simulink model "DFADAS2_SenFus_v1_201204RC_training_210115"  (R2018b)
settings: Solver=FixedStepDiscrete  StartTime=0.0  StopTime=inf  FixedStep=0.002  RelTol=1e-3  EnableMultiTasking=on
PreLoadFcn:
  | RTWConfigurationCB('preloadfcn', bdroot);
libraries: canmsglib x108, simulink x48, canfdmsglib x12
(part 5 of 28)

== system DFADAS2_SenFus_v1_201204RC_training_210115/Measure Calibration Debug/CAN Monitor (CANMon)/Subsystem1 ==
  <RLObj2> : Inport
  Bus Selector2 : BusSelector  OutputSignals=ID,Xpos,Ypos
  CAN Pack7 : canmsglib/CAN Pack  MsgList=(none)  MsgName=CAN Msg  MsgIDType=Standard (11-bit identifier)  MsgIdentifier=2033  MsgLength=8  SignalInfo=ID$0$16$1$2$1$0$1$0$-Inf$Inf$#Xpos$16$16$1$2$1$0$0.05$-400$-Inf$Inf$#Ypos$32$16$1$2$1$0$0.01$-80$-Inf$Inf$#  NSignals=3  StartBits=str2num('[int32(0);int32(16);int32(32)]')  SignalSizes=str2num('[int32(16);int32(16);int32(16)]')  ByteOrders=str2num('[int32(1);int32(1);int32(1)]')  DataTypes=str2num('[int32(2);int32(2);int32(2)]')  MultiplexTypes=str2num('[int32(1);int32(1);int32(1)]')  MultiplexValues=str2num('[double(0);double(0);double(0)]')  Factors=str2num('[double(1);double(0.05);double(0.01)]')  Offsets=str2num('[double(0);double(-400);double(-80)]')  Minimums=str2num('[double(-Inf);double(-Inf);double(-Inf)]')  Maximums=str2num('[double(Inf);double(Inf);double(Inf)]')  Remote=off  ApplyMinMax=off  BusOutput=on
      settings: SourceProductName=Simulink Real-Time  SourceProductBaseCode=XP  DataFormat=manually specified signals
  S-Function6 : S-Function  FunctionName=NSTC297CANTransmitBlkLib  Parameters=|  SFunctionDeploymentMode=off  EnableBusSupport=off  mask(NSTC297 CAN Transmit){Ns_DeviceID=General Control Unit Gen2, Ns_ChannelNum=0, Ns_FrameType=CAN, Ns_FrameBufferSize=0, Ns_OverflowCntOutFlg=off, Ns_SampleTime=-1}
      | uint16(Ns_DeviceID),
      | uint16(Ns_ChannelNum),
      | uint16(Ns_FrameType),
      | uint16(Ns_FrameBufferSize),
      | uint8(Ns_OverflowCntOutFlg),
      | double(Ns_SampleTime)
      mask prompts: Ns_DeviceID "Device:"; Ns_ChannelNum "Channel number:"; Ns_FrameType "Frame type:"; Ns_FrameBufferSize "Frame buffer size:"; Ns_OverflowCntOutFlg "Overflow count output"; Ns_SampleTime "Sample time:"
      mask init:
      | NSTC297CANTransmit_callback('portlabels');
      mask TypeOptions Ns_DeviceID: General Control Unit Gen2 | ADAS Control Unit Gen2
      mask TypeOptions Ns_ChannelNum: 0 | 1 | 2 | 3 | 4 | 5
      mask TypeOptions Ns_FrameType: CAN | CANFD
      mask Display: color('blue');text(0.98,0.9,'NovSteeds TC297','horizontalAlignment','right');color('blue');text(0.5,0.65,'CAN Transmit','horizontalAlignment','center');color('black');text(0.5,0.35,'Type: CAN','horizontalAlignment','center');text(0.5,0.50,'Channel: 0','horizontalAlignment','center');port_label('input',1, 'Msg');
  wires:
  CAN Pack7/1 -> S-Function6/1
  <RLObj2>/1 -> Bus Selector2/1
  Bus Selector2/2 -> CAN Pack7/2  "<Xpos>"
  Bus Selector2/3 -> CAN Pack7/3  "<Ypos>"
  Bus Selector2/1 -> CAN Pack7/1  "<ID>"

== system DFADAS2_SenFus_v1_201204RC_training_210115/Measure Calibration Debug/CAN Monitor (CANMon)/Subsystem2 ==
  <RLObj3> : Inport
  Bus Selector2 : BusSelector  OutputSignals=ID,Xpos,Ypos
  CAN Pack7 : canmsglib/CAN Pack  MsgList=(none)  MsgName=CAN Msg  MsgIDType=Standard (11-bit identifier)  MsgIdentifier=2034  MsgLength=8  SignalInfo=ID$0$16$1$2$1$0$1$0$-Inf$Inf$#Xpos$16$16$1$2$1$0$0.05$-400$-Inf$Inf$#Ypos$32$16$1$2$1$0$0.01$-80$-Inf$Inf$#  NSignals=3  StartBits=str2num('[int32(0);int32(16);int32(32)]')  SignalSizes=str2num('[int32(16);int32(16);int32(16)]')  ByteOrders=str2num('[int32(1);int32(1);int32(1)]')  DataTypes=str2num('[int32(2);int32(2);int32(2)]')  MultiplexTypes=str2num('[int32(1);int32(1);int32(1)]')  MultiplexValues=str2num('[double(0);double(0);double(0)]')  Factors=str2num('[double(1);double(0.05);double(0.01)]')  Offsets=str2num('[double(0);double(-400);double(-80)]')  Minimums=str2num('[double(-Inf);double(-Inf);double(-Inf)]')  Maximums=str2num('[double(Inf);double(Inf);double(Inf)]')  Remote=off  ApplyMinMax=off  BusOutput=on
      settings: SourceProductName=Simulink Real-Time  SourceProductBaseCode=XP  DataFormat=manually specified signals
  S-Function6 : S-Function  FunctionName=NSTC297CANTransmitBlkLib  Parameters=|  SFunctionDeploymentMode=off  EnableBusSupport=off  mask(NSTC297 CAN Transmit){Ns_DeviceID=General Control Unit Gen2, Ns_ChannelNum=0, Ns_FrameType=CAN, Ns_FrameBufferSize=0, Ns_OverflowCntOutFlg=off, Ns_SampleTime=-1}
      | uint16(Ns_DeviceID),
      | uint16(Ns_ChannelNum),
      | uint16(Ns_FrameType),
      | uint16(Ns_FrameBufferSize),
      | uint8(Ns_OverflowCntOutFlg),
      | double(Ns_SampleTime)
      mask prompts: Ns_DeviceID "Device:"; Ns_ChannelNum "Channel number:"; Ns_FrameType "Frame type:"; Ns_FrameBufferSize "Frame buffer size:"; Ns_OverflowCntOutFlg "Overflow count output"; Ns_SampleTime "Sample time:"
      mask init:
      | NSTC297CANTransmit_callback('portlabels');
      mask TypeOptions Ns_DeviceID: General Control Unit Gen2 | ADAS Control Unit Gen2
      mask TypeOptions Ns_ChannelNum: 0 | 1 | 2 | 3 | 4 | 5
      mask TypeOptions Ns_FrameType: CAN | CANFD
      mask Display: color('blue');text(0.98,0.9,'NovSteeds TC297','horizontalAlignment','right');color('blue');text(0.5,0.65,'CAN Transmit','horizontalAlignment','center');color('black');text(0.5,0.35,'Type: CAN','horizontalAlignment','center');text(0.5,0.50,'Channel: 0','horizontalAlignment','center');port_label('input',1, 'Msg');
  wires:
  CAN Pack7/1 -> S-Function6/1
  <RLObj3>/1 -> Bus Selector2/1
  Bus Selector2/2 -> CAN Pack7/2  "<Xpos>"
  Bus Selector2/3 -> CAN Pack7/3  "<Ypos>"
  Bus Selector2/1 -> CAN Pack7/1  "<ID>"

== system DFADAS2_SenFus_v1_201204RC_training_210115/Measure Calibration Debug/CAN Monitor (CANMon)/Subsystem3 ==
  <RLObj4> : Inport
  Bus Selector2 : BusSelector  OutputSignals=ID,Xpos,Ypos
  CAN Pack7 : canmsglib/CAN Pack  MsgList=(none)  MsgName=CAN Msg  MsgIDType=Standard (11-bit identifier)  MsgIdentifier=2035  MsgLength=8  SignalInfo=ID$0$16$1$2$1$0$1$0$-Inf$Inf$#Xpos$16$16$1$2$1$0$0.05$-400$-Inf$Inf$#Ypos$32$16$1$2$1$0$0.01$-80$-Inf$Inf$#  NSignals=3  StartBits=str2num('[int32(0);int32(16);int32(32)]')  SignalSizes=str2num('[int32(16);int32(16);int32(16)]')  ByteOrders=str2num('[int32(1);int32(1);int32(1)]')  DataTypes=str2num('[int32(2);int32(2);int32(2)]')  MultiplexTypes=str2num('[int32(1);int32(1);int32(1)]')  MultiplexValues=str2num('[double(0);double(0);double(0)]')  Factors=str2num('[double(1);double(0.05);double(0.01)]')  Offsets=str2num('[double(0);double(-400);double(-80)]')  Minimums=str2num('[double(-Inf);double(-Inf);double(-Inf)]')  Maximums=str2num('[double(Inf);double(Inf);double(Inf)]')  Remote=off  ApplyMinMax=off  BusOutput=on
      settings: SourceProductName=Simulink Real-Time  SourceProductBaseCode=XP  DataFormat=manually specified signals
  S-Function6 : S-Function  FunctionName=NSTC297CANTransmitBlkLib  Parameters=|  SFunctionDeploymentMode=off  EnableBusSupport=off  mask(NSTC297 CAN Transmit){Ns_DeviceID=General Control Unit Gen2, Ns_ChannelNum=0, Ns_FrameType=CAN, Ns_FrameBufferSize=0, Ns_OverflowCntOutFlg=off, Ns_SampleTime=-1}
      | uint16(Ns_DeviceID),
      | uint16(Ns_ChannelNum),
      | uint16(Ns_FrameType),
      | uint16(Ns_FrameBufferSize),
      | uint8(Ns_OverflowCntOutFlg),
      | double(Ns_SampleTime)
      mask prompts: Ns_DeviceID "Device:"; Ns_ChannelNum "Channel number:"; Ns_FrameType "Frame type:"; Ns_FrameBufferSize "Frame buffer size:"; Ns_OverflowCntOutFlg "Overflow count output"; Ns_SampleTime "Sample time:"
      mask init:
      | NSTC297CANTransmit_callback('portlabels');
      mask TypeOptions Ns_DeviceID: General Control Unit Gen2 | ADAS Control Unit Gen2
      mask TypeOptions Ns_ChannelNum: 0 | 1 | 2 | 3 | 4 | 5
      mask TypeOptions Ns_FrameType: CAN | CANFD
      mask Display: color('blue');text(0.98,0.9,'NovSteeds TC297','horizontalAlignment','right');color('blue');text(0.5,0.65,'CAN Transmit','horizontalAlignment','center');color('black');text(0.5,0.35,'Type: CAN','horizontalAlignment','center');text(0.5,0.50,'Channel: 0','horizontalAlignment','center');port_label('input',1, 'Msg');
  wires:
  Bus Selector2/1 -> CAN Pack7/1  "<ID>"
  Bus Selector2/3 -> CAN Pack7/3  "<Ypos>"
  Bus Selector2/2 -> CAN Pack7/2  "<Xpos>"
  <RLObj4>/1 -> Bus Selector2/1
  CAN Pack7/1 -> S-Function6/1

== system DFADAS2_SenFus_v1_201204RC_training_210115/Measure Calibration Debug/CAN Monitor (CANMon)/Subsystem4 ==
  <RLObj5> : Inport
  Bus Selector2 : BusSelector  OutputSignals=ID,Xpos,Ypos
  CAN Pack7 : canmsglib/CAN Pack  MsgList=(none)  MsgName=CAN Msg  MsgIDType=Standard (11-bit identifier)  MsgIdentifier=2036  MsgLength=8  SignalInfo=ID$0$16$1$2$1$0$1$0$-Inf$Inf$#Xpos$16$16$1$2$1$0$0.05$-400$-Inf$Inf$#Ypos$32$16$1$2$1$0$0.01$-80$-Inf$Inf$#  NSignals=3  StartBits=str2num('[int32(0);int32(16);int32(32)]')  SignalSizes=str2num('[int32(16);int32(16);int32(16)]')  ByteOrders=str2num('[int32(1);int32(1);int32(1)]')  DataTypes=str2num('[int32(2);int32(2);int32(2)]')  MultiplexTypes=str2num('[int32(1);int32(1);int32(1)]')  MultiplexValues=str2num('[double(0);double(0);double(0)]')  Factors=str2num('[double(1);double(0.05);double(0.01)]')  Offsets=str2num('[double(0);double(-400);double(-80)]')  Minimums=str2num('[double(-Inf);double(-Inf);double(-Inf)]')  Maximums=str2num('[double(Inf);double(Inf);double(Inf)]')  Remote=off  ApplyMinMax=off  BusOutput=on
      settings: SourceProductName=Simulink Real-Time  SourceProductBaseCode=XP  DataFormat=manually specified signals
  S-Function6 : S-Function  FunctionName=NSTC297CANTransmitBlkLib  Parameters=|  SFunctionDeploymentMode=off  EnableBusSupport=off  mask(NSTC297 CAN Transmit){Ns_DeviceID=General Control Unit Gen2, Ns_ChannelNum=0, Ns_FrameType=CAN, Ns_FrameBufferSize=0, Ns_OverflowCntOutFlg=off, Ns_SampleTime=-1}
      | uint16(Ns_DeviceID),
      | uint16(Ns_ChannelNum),
      | uint16(Ns_FrameType),
      | uint16(Ns_FrameBufferSize),
      | uint8(Ns_OverflowCntOutFlg),
      | double(Ns_SampleTime)
      mask prompts: Ns_DeviceID "Device:"; Ns_ChannelNum "Channel number:"; Ns_FrameType "Frame type:"; Ns_FrameBufferSize "Frame buffer size:"; Ns_OverflowCntOutFlg "Overflow count output"; Ns_SampleTime "Sample time:"
      mask init:
      | NSTC297CANTransmit_callback('portlabels');
      mask TypeOptions Ns_DeviceID: General Control Unit Gen2 | ADAS Control Unit Gen2
      mask TypeOptions Ns_ChannelNum: 0 | 1 | 2 | 3 | 4 | 5
      mask TypeOptions Ns_FrameType: CAN | CANFD
      mask Display: color('blue');text(0.98,0.9,'NovSteeds TC297','horizontalAlignment','right');color('blue');text(0.5,0.65,'CAN Transmit','horizontalAlignment','center');color('black');text(0.5,0.35,'Type: CAN','horizontalAlignment','center');text(0.5,0.50,'Channel: 0','horizontalAlignment','center');port_label('input',1, 'Msg');
  wires:
  CAN Pack7/1 -> S-Function6/1
  <RLObj5>/1 -> Bus Selector2/1
  Bus Selector2/2 -> CAN Pack7/2  "<Xpos>"
  Bus Selector2/3 -> CAN Pack7/3  "<Ypos>"
  Bus Selector2/1 -> CAN Pack7/1  "<ID>"

== system DFADAS2_SenFus_v1_201204RC_training_210115/Measure Calibration Debug/CAN Monitor (CANMon)/Subsystem5 ==
  <RLObj6> : Inport
  Bus Selector2 : BusSelector  OutputSignals=ID,Xpos,Ypos
  CAN Pack7 : canmsglib/CAN Pack  MsgList=(none)  MsgName=CAN Msg  MsgIDType=Standard (11-bit identifier)  MsgIdentifier=2037  MsgLength=8  SignalInfo=ID$0$16$1$2$1$0$1$0$-Inf$Inf$#Xpos$16$16$1$2$1$0$0.05$-400$-Inf$Inf$#Ypos$32$16$1$2$1$0$0.01$-80$-Inf$Inf$#  NSignals=3  StartBits=str2num('[int32(0);int32(16);int32(32)]')  SignalSizes=str2num('[int32(16);int32(16);int32(16)]')  ByteOrders=str2num('[int32(1);int32(1);int32(1)]')  DataTypes=str2num('[int32(2);int32(2);int32(2)]')  MultiplexTypes=str2num('[int32(1);int32(1);int32(1)]')  MultiplexValues=str2num('[double(0);double(0);double(0)]')  Factors=str2num('[double(1);double(0.05);double(0.01)]')  Offsets=str2num('[double(0);double(-400);double(-80)]')  Minimums=str2num('[double(-Inf);double(-Inf);double(-Inf)]')  Maximums=str2num('[double(Inf);double(Inf);double(Inf)]')  Remote=off  ApplyMinMax=off  BusOutput=on
      settings: SourceProductName=Simulink Real-Time  SourceProductBaseCode=XP  DataFormat=manually specified signals
  S-Function6 : S-Function  FunctionName=NSTC297CANTransmitBlkLib  Parameters=|  SFunctionDeploymentMode=off  EnableBusSupport=off  mask(NSTC297 CAN Transmit){Ns_DeviceID=General Control Unit Gen2, Ns_ChannelNum=0, Ns_FrameType=CAN, Ns_FrameBufferSize=0, Ns_OverflowCntOutFlg=off, Ns_SampleTime=-1}
      | uint16(Ns_DeviceID),
      | uint16(Ns_ChannelNum),
      | uint16(Ns_FrameType),
      | uint16(Ns_FrameBufferSize),
      | uint8(Ns_OverflowCntOutFlg),
      | double(Ns_SampleTime)
      mask prompts: Ns_DeviceID "Device:"; Ns_ChannelNum "Channel number:"; Ns_FrameType "Frame type:"; Ns_FrameBufferSize "Frame buffer size:"; Ns_OverflowCntOutFlg "Overflow count output"; Ns_SampleTime "Sample time:"
      mask init:
      | NSTC297CANTransmit_callback('portlabels');
      mask TypeOptions Ns_DeviceID: General Control Unit Gen2 | ADAS Control Unit Gen2
      mask TypeOptions Ns_ChannelNum: 0 | 1 | 2 | 3 | 4 | 5
      mask TypeOptions Ns_FrameType: CAN | CANFD
      mask Display: color('blue');text(0.98,0.9,'NovSteeds TC297','horizontalAlignment','right');color('blue');text(0.5,0.65,'CAN Transmit','horizontalAlignment','center');color('black');text(0.5,0.35,'Type: CAN','horizontalAlignment','center');text(0.5,0.50,'Channel: 0','horizontalAlignment','center');port_label('input',1, 'Msg');
  wires:
  Bus Selector2/1 -> CAN Pack7/1  "<ID>"
  Bus Selector2/3 -> CAN Pack7/3  "<Ypos>"
  Bus Selector2/2 -> CAN Pack7/2  "<Xpos>"
  <RLObj6>/1 -> Bus Selector2/1
  CAN Pack7/1 -> S-Function6/1

== system DFADAS2_SenFus_v1_201204RC_training_210115/Measure Calibration Debug/CAN Monitor (CANMon)/Subsystem6 ==
  <RLObj7> : Inport
  Bus Selector2 : BusSelector  OutputSignals=ID,Xpos,Ypos
  CAN Pack7 : canmsglib/CAN Pack  MsgList=(none)  MsgName=CAN Msg  MsgIDType=Standard (11-bit identifier)  MsgIdentifier=2038  MsgLength=8  SignalInfo=ID$0$16$1$2$1$0$1$0$-Inf$Inf$#Xpos$16$16$1$2$1$0$0.05$-400$-Inf$Inf$#Ypos$32$16$1$2$1$0$0.01$-80$-Inf$Inf$#  NSignals=3  StartBits=str2num('[int32(0);int32(16);int32(32)]')  SignalSizes=str2num('[int32(16);int32(16);int32(16)]')  ByteOrders=str2num('[int32(1);int32(1);int32(1)]')  DataTypes=str2num('[int32(2);int32(2);int32(2)]')  MultiplexTypes=str2num('[int32(1);int32(1);int32(1)]')  MultiplexValues=str2num('[double(0);double(0);double(0)]')  Factors=str2num('[double(1);double(0.05);double(0.01)]')  Offsets=str2num('[double(0);double(-400);double(-80)]')  Minimums=str2num('[double(-Inf);double(-Inf);double(-Inf)]')  Maximums=str2num('[double(Inf);double(Inf);double(Inf)]')  Remote=off  ApplyMinMax=off  BusOutput=on
      settings: SourceProductName=Simulink Real-Time  SourceProductBaseCode=XP  DataFormat=manually specified signals
  S-Function6 : S-Function  FunctionName=NSTC297CANTransmitBlkLib  Parameters=|  SFunctionDeploymentMode=off  EnableBusSupport=off  mask(NSTC297 CAN Transmit){Ns_DeviceID=General Control Unit Gen2, Ns_ChannelNum=0, Ns_FrameType=CAN, Ns_FrameBufferSize=0, Ns_OverflowCntOutFlg=off, Ns_SampleTime=-1}
      | uint16(Ns_DeviceID),
      | uint16(Ns_ChannelNum),
      | uint16(Ns_FrameType),
      | uint16(Ns_FrameBufferSize),
      | uint8(Ns_OverflowCntOutFlg),
      | double(Ns_SampleTime)
      mask prompts: Ns_DeviceID "Device:"; Ns_ChannelNum "Channel number:"; Ns_FrameType "Frame type:"; Ns_FrameBufferSize "Frame buffer size:"; Ns_OverflowCntOutFlg "Overflow count output"; Ns_SampleTime "Sample time:"
      mask init:
      | NSTC297CANTransmit_callback('portlabels');
      mask TypeOptions Ns_DeviceID: General Control Unit Gen2 | ADAS Control Unit Gen2
      mask TypeOptions Ns_ChannelNum: 0 | 1 | 2 | 3 | 4 | 5
      mask TypeOptions Ns_FrameType: CAN | CANFD
      mask Display: color('blue');text(0.98,0.9,'NovSteeds TC297','horizontalAlignment','right');color('blue');text(0.5,0.65,'CAN Transmit','horizontalAlignment','center');color('black');text(0.5,0.35,'Type: CAN','horizontalAlignment','center');text(0.5,0.50,'Channel: 0','horizontalAlignment','center');port_label('input',1, 'Msg');
  wires:
  Bus Selector2/1 -> CAN Pack7/1  "<ID>"
  Bus Selector2/3 -> CAN Pack7/3  "<Ypos>"
  Bus Selector2/2 -> CAN Pack7/2  "<Xpos>"
  <RLObj7>/1 -> Bus Selector2/1
  CAN Pack7/1 -> S-Function6/1

== system DFADAS2_SenFus_v1_201204RC_training_210115/Measure Calibration Debug/CAN Monitor (CANMon)/Subsystem7 ==
  <RLObj8> : Inport
  Bus Selector2 : BusSelector  OutputSignals=ID,Xpos,Ypos
  CAN Pack7 : canmsglib/CAN Pack  MsgList=(none)  MsgName=CAN Msg  MsgIDType=Standard (11-bit identifier)  MsgIdentifier=2039  MsgLength=8  SignalInfo=ID$0$16$1$2$1$0$1$0$-Inf$Inf$#Xpos$16$16$1$2$1$0$0.05$-400$-Inf$Inf$#Ypos$32$16$1$2$1$0$0.01$-80$-Inf$Inf$#  NSignals=3  StartBits=str2num('[int32(0);int32(16);int32(32)]')  SignalSizes=str2num('[int32(16);int32(16);int32(16)]')  ByteOrders=str2num('[int32(1);int32(1);int32(1)]')  DataTypes=str2num('[int32(2);int32(2);int32(2)]')  MultiplexTypes=str2num('[int32(1);int32(1);int32(1)]')  MultiplexValues=str2num('[double(0);double(0);double(0)]')  Factors=str2num('[double(1);double(0.05);double(0.01)]')  Offsets=str2num('[double(0);double(-400);double(-80)]')  Minimums=str2num('[double(-Inf);double(-Inf);double(-Inf)]')  Maximums=str2num('[double(Inf);double(Inf);double(Inf)]')  Remote=off  ApplyMinMax=off  BusOutput=on
      settings: SourceProductName=Simulink Real-Time  SourceProductBaseCode=XP  DataFormat=manually specified signals
  S-Function6 : S-Function  FunctionName=NSTC297CANTransmitBlkLib  Parameters=|  SFunctionDeploymentMode=off  EnableBusSupport=off  mask(NSTC297 CAN Transmit){Ns_DeviceID=General Control Unit Gen2, Ns_ChannelNum=0, Ns_FrameType=CAN, Ns_FrameBufferSize=0, Ns_OverflowCntOutFlg=off, Ns_SampleTime=-1}
      | uint16(Ns_DeviceID),
      | uint16(Ns_ChannelNum),
      | uint16(Ns_FrameType),
      | uint16(Ns_FrameBufferSize),
      | uint8(Ns_OverflowCntOutFlg),
      | double(Ns_SampleTime)
      mask prompts: Ns_DeviceID "Device:"; Ns_ChannelNum "Channel number:"; Ns_FrameType "Frame type:"; Ns_FrameBufferSize "Frame buffer size:"; Ns_OverflowCntOutFlg "Overflow count output"; Ns_SampleTime "Sample time:"
      mask init:
      | NSTC297CANTransmit_callback('portlabels');
      mask TypeOptions Ns_DeviceID: General Control Unit Gen2 | ADAS Control Unit Gen2
      mask TypeOptions Ns_ChannelNum: 0 | 1 | 2 | 3 | 4 | 5
      mask TypeOptions Ns_FrameType: CAN | CANFD
      mask Display: color('blue');text(0.98,0.9,'NovSteeds TC297','horizontalAlignment','right');color('blue');text(0.5,0.65,'CAN Transmit','horizontalAlignment','center');color('black');text(0.5,0.35,'Type: CAN','horizontalAlignment','center');text(0.5,0.50,'Channel: 0','horizontalAlignment','center');port_label('input',1, 'Msg');
  wires:
  CAN Pack7/1 -> S-Function6/1
  <RLObj8>/1 -> Bus Selector2/1
  Bus Selector2/2 -> CAN Pack7/2  "<Xpos>"
  Bus Selector2/3 -> CAN Pack7/3  "<Ypos>"
  Bus Selector2/1 -> CAN Pack7/1  "<ID>"

== system DFADAS2_SenFus_v1_201204RC_training_210115/Signal Input (Input)/Signal Input (10ms) (Input10)/Others ==
  Bus Creator1 : BusCreator  Inputs=3
  Constant4 : Constant  Value=0.3
  Constant5 : Constant  Value=0.3
  Constant6 : Constant  Value=0.3
  Out1 : Outport
  wires:
  Bus Creator1/1 -> Out1/1  "VehInfo"
  Constant6/1 -> Bus Creator1/3
  Constant5/1 -> Bus Creator1/2
  Constant4/1 -> Bus Creator1/1

== system DFADAS2_SenFus_v1_201204RC_training_210115/Signal Input (Input)/Signal Input (10ms) (Input10)/VehInfo ==
  note: Level: 2
  ACC_AdditionalSignal_1 : Subsystem
  ACC_AdditionalSignal_20190523 : Subsystem
  Body Electric System State Receive and Processing (BESRx) : Subsystem
  Bus Creator2 : BusCreator  Inputs=10
  EPS Signal Receive and Processing (EPSRx) : Subsystem
  "ForwardVeh_sigback " : Subsystem
  From ACC (From ACC) : Subsystem
  Function Keys State Receive and Processing (FKeyStRx) : Subsystem
  MP5 Signal Receive (MP5Rx)1 : Subsystem
  Powertrain State Receive and Processing (PTRx) : Subsystem
  Steeing Wheel Angle Receive and Processing (SWARx) : Subsystem
  Vehicle Movement Signal Receive and Processing (VehMovRx) : Subsystem
  VehInfo : Outport
  tag scope: Acc_DisplaySig=global
  wires:
  Bus Creator2/1 -> VehInfo/1  "bsVehInfo"
  ACC_AdditionalSignal_1/1(Acc_DisplaySig) -> [Acc_DisplaySig]
  MP5 Signal Receive (MP5Rx)1/1(MP5Rx_bsMP5Info) -> Bus Creator2/1  "MP5Rx_bsMP5Info"
  EPS Signal Receive and Processing (EPSRx)/1(EPSRx_bsEPSInfo) -> Bus Creator2/2  "EPSRx_bsEPSInfo"
  Vehicle Movement Signal Receive and Processing (VehMovRx)/1(VehMovRx_bsVehMovInfo) -> Bus Creator2/3  "VehMovRx_bsVehMovInfo"
  Steeing Wheel Angle Receive and Processing (SWARx)/1(SWARx_bsSWAInfo) -> Bus Creator2/4  "SWARx_bsSWAInfo"
  Body Electric System State Receive and Processing (BESRx)/1(BESRx_bsBESState) -> Bus Creator2/5  "BESRx_bsBESState"
  Function Keys State Receive and Processing (FKeyStRx)/1(FKeyStRx_stFKeyState) -> Bus Creator2/6  "FKeyStRx_stFKeyState"
  Powertrain State Receive and Processing (PTRx)/1(PTRx_bsPTState) -> Bus Creator2/7  "PTRx_bsPTState"
  From ACC (From ACC)/1(From ACC_stACCState) -> Bus Creator2/8  "From ACC_stACCState"
  ACC_AdditionalSignal_20190523/1(DACIn_bsACCAdditionalSignal) -> Bus Creator2/9  "FMCRx_ACCAdditionalSignal"
  "ForwardVeh_sigback "/1(SpdReq_bsSpdDet1info) -> Bus Creator2/10  "SpdReq_bsSpdDet1info"

== system DFADAS2_SenFus_v1_201204RC_training_210115/Signal Input (Input)/Signal Input (50ms) (Input50)/Cmr ==
  note: Device Signal Level
  Camera Objects Information (CmrObjInfo) : Subsystem
  CmrInfo : Subsystem
  Cmr_bsComInfo : Outport
  Cmr_bsTrafSig : Outport  Port=2
  Cmr_bsObjInfo : Outport  Port=3
  wires:
  Camera Objects Information (CmrObjInfo)/1(CmrObjRx_bsObjInfo) -> Cmr_bsObjInfo/1  "CmrObjInfo"
  CmrInfo/1(LaneRx_bsLaneInfo) -> Cmr_bsComInfo/1  "LaneInfo"

== system DFADAS2_SenFus_v1_201204RC_training_210115/Signal Input (Input)/Signal Input (50ms) (Input50)/Front Left Radar(S2) Objects Information (FLRdr) ==
  Bus Creator : BusCreator  Inputs=2
  Bus Selector : BusSelector  OutputSignals=NumberOfObjects_S2
  Constant1 : Constant  SampleTime=0.05
  Constant2 : Constant  SampleTime=0.05
  Constant3 : Constant  SampleTime=0.05
  S0 Data Frame Read : Subsystem  TreatAsAtomicUnit=on
  S0 Header Frame Read : Subsystem  TreatAsAtomicUnit=on
  S0 Trailer Frame Read : Subsystem  TreatAsAtomicUnit=on
  Subsystem : Subsystem  Commented=on
  FLRdr_bsObjInfo : Outport
  wires:
  Bus Creator/1 -> FLRdr_bsObjInfo/1, Subsystem/1(In1)
  Bus Selector/1 -> S0 Data Frame Read/3(ObjectNum)  "<NumberOfObjects_S2>"
  S0 Header Frame Read/1(RLRdr_bsCmnInfo) -> Bus Selector/1, Bus Creator/1  "FLRdr_bsCmnInfo"
  S0 Data Frame Read/1(RLRdr_bsObjInfo) -> Bus Creator/2  "FLRdr_bsObjInfo"
  Constant2/1 -> S0 Data Frame Read/2(IC)
  Constant1/1 -> S0 Trailer Frame Read/2("IC ")
  Constant3/1 -> S0 Header Frame Read/1(IC)
  S0 Header Frame Read/2(HFVFCnt) -> S0 Data Frame Read/1(HFVFCnt), S0 Trailer Frame Read/1(HFVFCnt)

== system DFADAS2_SenFus_v1_201204RC_training_210115/Signal Input (Input)/Signal Input (50ms) (Input50)/Front Right Radar(S3) Objects Information (FRRdr) ==
  Bus Creator : BusCreator  Inputs=2
  Bus Selector : BusSelector  OutputSignals=NumberOfObjects_S3
  Constant1 : Constant  SampleTime=0.05
  Constant2 : Constant  SampleTime=0.05
  Constant3 : Constant  SampleTime=0.05
  S0 Data Frame Read : Subsystem  TreatAsAtomicUnit=on
  S0 Header Frame Read : Subsystem  TreatAsAtomicUnit=on
  S0 Trailer Frame Read : Subsystem  TreatAsAtomicUnit=on
  Subsystem : Subsystem  Commented=on
  FRRdr_bsObjInfo : Outport
  wires:
  Bus Creator/1 -> FRRdr_bsObjInfo/1, Subsystem/1(In1)
  S0 Data Frame Read/1(RLRdr_bsObjInfo) -> Bus Creator/2  "FRRdr_bsObjInfo"
  S0 Header Frame Read/2(HFVFCnt) -> S0 Trailer Frame Read/1(HFVFCnt), S0 Data Frame Read/1(HFVFCnt)
  Constant3/1 -> S0 Header Frame Read/1(IC)
  Constant1/1 -> S0 Trailer Frame Read/2("IC ")
  Constant2/1 -> S0 Data Frame Read/2(IC)
  S0 Header Frame Read/1(RLRdr_bsCmnInfo) -> Bus Selector/1, Bus Creator/1  "FRRdr_bsCmnInfo"
  Bus Selector/1 -> S0 Data Frame Read/3(ObjectNum)  "<NumberOfObjects_S3>"

== system DFADAS2_SenFus_v1_201204RC_training_210115/Signal Input (Input)/Signal Input (50ms) (Input50)/Others ==
  Bus Creator1 : BusCreator  Inputs=3
  Constant4 : Constant  Value=0.3
  Constant5 : Constant  Value=0.3
  Constant6 : Constant  Value=0.3
  Out1 : Outport
  wires:
  Bus Creator1/1 -> Out1/1  "VehInfo"
  Constant6/1 -> Bus Creator1/3
  Constant5/1 -> Bus Creator1/2
  Constant4/1 -> Bus Creator1/1

== system DFADAS2_SenFus_v1_201204RC_training_210115/Signal Input (Input)/Signal Input (50ms) (Input50)/RdrFrt ==
  note: ① 设备：完整性
      | ② 信号及状态
  note: 首先按设备分层；然后按功能对信号聚类与分层。
  Bus Creator1 : BusCreator  Inputs=2
  CmrInfo : Subsystem
  Rdr1 : Subsystem
  Out1 : Outport
  wires:
  Bus Creator1/1 -> Out1/1
  Rdr1/1(Out1) -> Bus Creator1/2
  CmrInfo/1(Out1) -> Bus Creator1/1

== system DFADAS2_SenFus_v1_201204RC_training_210115/Signal Input (Input)/Signal Input (50ms) (Input50)/Rear Left Radar(S0) Objects Information (RLRdr) ==
  Bus Creator : BusCreator  Inputs=2
  Bus Selector : BusSelector  OutputSignals=NumberOfObjects_S0
  Constant1 : Constant  SampleTime=0.05
  Constant2 : Constant  SampleTime=0.05
  Constant3 : Constant  SampleTime=0.05
  S0 Data Frame Read : Subsystem  TreatAsAtomicUnit=on
  S0 Header Frame Read : Subsystem  TreatAsAtomicUnit=on
  S0 Trailer Frame Read : Subsystem  TreatAsAtomicUnit=on
  Subsystem : Subsystem  Commented=on
  RLRdr_bsObjInfo : Outport
  wires:
  S0 Header Frame Read/2(HFVFCnt) -> S0 Trailer Frame Read/1(HFVFCnt), S0 Data Frame Read/1(HFVFCnt)
  Constant3/1 -> S0 Header Frame Read/1(IC)
  Constant1/1 -> S0 Trailer Frame Read/2("IC ")
  Constant2/1 -> S0 Data Frame Read/2(IC)
  S0 Data Frame Read/1(RLRdr_bsObjInfo) -> Bus Creator/2  "RLRdr_bsObjInfo"
  S0 Header Frame Read/1(RLRdr_bsCmnInfo) -> Bus Creator/1, Bus Selector/1  "RLRdr_bsCmnInfo"
  Bus Selector/1 -> S0 Data Frame Read/3(ObjectNum)  "<NumberOfObjects_S0>"
  Bus Creator/1 -> Subsystem/1(In1), RLRdr_bsObjInfo/1

== system DFADAS2_SenFus_v1_201204RC_training_210115/Signal Input (Input)/Signal Input (50ms) (Input50)/Rear Right Radar(S1) Objects Information (RRRdr) ==
  Bus Creator : BusCreator  Inputs=2
  Bus Selector : BusSelector  OutputSignals=NumberOfObjects_S1
  Constant1 : Constant  SampleTime=0.05
  Constant2 : Constant  SampleTime=0.05
  Constant3 : Constant  SampleTime=0.05
  S0 Data Frame Read : Subsystem  TreatAsAtomicUnit=on
  S0 Header Frame Read : Subsystem  TreatAsAtomicUnit=on
  S0 Trailer Frame Read : Subsystem  TreatAsAtomicUnit=on
  Subsystem : Subsystem  Commented=on
  RRRdr_bsObjInfo : Outport
  wires:
  Bus Selector/1 -> S0 Data Frame Read/3(ObjectNum)  "<NumberOfObjects_S1>"
  S0 Header Frame Read/1(RLRdr_bsCmnInfo) -> Bus Creator/1, Bus Selector/1  "RRRdr_bsCmnInfo"
  Constant2/1 -> S0 Data Frame Read/2(IC)
  Constant1/1 -> S0 Trailer Frame Read/2("IC ")
  Constant3/1 -> S0 Header Frame Read/1(IC)
  S0 Header Frame Read/2(HFVFCnt) -> S0 Data Frame Read/1(HFVFCnt), S0 Trailer Frame Read/1(HFVFCnt)
  S0 Data Frame Read/1(RLRdr_bsObjInfo) -> Bus Creator/2  "RRRdr_bsObjInfo"
  Bus Creator/1 -> Subsystem/1(In1), RRRdr_bsObjInfo/1

== system DFADAS2_SenFus_v1_201204RC_training_210115/Signal Input (Input)/Signal Input (10ms) (Input10)/VehInfo/ACC_AdditionalSignal_1 ==
  Bus Creator : BusCreator  Inputs=13
  CAN Unpack2 : canmsglib/CAN Unpack  CANdbFile=D:\document_ljj\2020_7\ADAS_ECU_PSA1_CAN_V2_v20190520.dbc  MsgList=ADAS_4F7_PSA1  MsgName=ADAS_4F7_PSA1  MsgIDType=Standard (11-bit identifier)  MsgIdentifier=667  MsgLength=8  SignalInfo=ACC_DesiredHeadway_Display$5$2$2$2$1$0$1$0$0$3$#ACC_DesiredHeadway_Icon_Basic$3$1$2$2$1$0$1$0$0$1$#ACC_Desired_Set_Speed$16$8$2$2$1$0$1$0$0$254$#ACC_Pop_Up_Message$8$4$2$2$1$0$1$0$0$15$#ACC_Set_Speed_Display$0$3$2$2$1$0$1$0$0$7$#ACC_Vehicle_Icon_Display$40$3$2$2$1$0$1$0$0$7$#AEB_Alert_Req$14$2$2$2$1$0$1$1$1$4$#AEB_Fault_Status$27$2$2$2$1$0$1$1$1$3$#AEB_Switch_Status$12$2$2$2$1$0$1$1$1$4$#AEB_tips$24$3$2$2$1$0$1$0$0$7$#ICA_HMI_Txt_Disp$32$4$2$2$1$0$1$0$0$15$#RVVACC_Vehiclespeed_request_type$7$1$2$2$1$0$1$0$0$1$#TJA_status_icon$38$2$2$2$1$0$1$0$0$3$#  NSignals=13  IDPort=off  TimestampPort=off  ErrorPort=off  RemotePort=off  LengthPort=off  StatusPort=off  StartBits=str2num('[int32(5);int32(3);int32(16);int32(8);int32(0);int32(40);int32(14);int32(27);int32(12);int32(24);int32(32);int32(7);int32(38)]')  SignalSizes=str2num('[int32(2);int32(1);int32(8);int32(4);int32(3);int32(3);int32(2);int32(2);int32(2);int32(3);int32(4);int32(1);int32(2)]')  ByteOrders=str2num('[int32(2);int32(2);int32(2);int32(2);int32(2);int32(2);int32(2);int32(2);int32(2);int32(2);int32(2);int32(2);int32(2)]')  DataTypes=str2num('[int32(2);int32(2);int32(2);int32(2);int32(2);int32(2);int32(2);int32(2);int32(2);int32(2);int32(2);int32(2);int32(2)]')  MultiplexTypes=str2num('[int32(1);int32(1);int32(1);int32(1);int32(1);int32(1);int32(1);int32(1);int32(1);int32(1);int32(1);int32(1);int32(1)]')  MultiplexValues=str2num('[double(0);double(0);double(0);double(0);double(0);double(0);double(0);double(0);double(0);double(0);double(0);double(0);double(0)]')  Factors=str2num('[double(1);double(1);double(1);double(1);double(1);double(1);double(1);double(1);double(1);double(1);double(1);double(1);double(1)]')  Offsets=str2num('[double(0);double(0);double(0);double(0);double(0);double(0);double(1);double(1);double(1);double(0);double(0);double(0);double(0)]')  Minimums=str2num('[double(0);double(0);double(0);double(0);double(0);double(0);double(1);double(1);double(1);double(0);double(0);double(0);double(0)]')  Maximums=str2num('[double(3);double(1);double(254);double(15);double(7);double(7);double(4);double(3);double(4);double(7);double(15);double(1);double(3)]')  ApplyMinMax=off
      settings: SourceProductName=Simulink Real-Time  SourceProductBaseCode=XP
  S-Function11 : S-Function  FunctionName=NSTC297CANReceiveBlkLib  Parameters=|  SFunctionDeploymentMode=off  EnableBusSupport=off  mask(NSTC297 CAN Receive){Ns_DeviceID=ADAS Control Unit Gen2, Ns_ChannelNum=4, Ns_FrameID=667, Ns_IsVirtualFrame=off, Ns_RoleInVirtualFrame=Header Frame, Ns_HeaderFrameID=0, Ns_VirtualFrameStatusFlg=off, Ns_IncompleteFrameCntFlg=off, Ns_OverflowCntFlg=off, Ns_FrameBufferSize=1, Ns_SampleTime=0.01}
      | uint16(Ns_DeviceID),
      | uint16(Ns_ChannelNum),
      | uint32(Ns_FrameID),
      | uint8(Ns_IsVirtualFrame),
      | uint16(Ns_RoleInVirtualFrame),
      | uint32(Ns_HeaderFrameID),
      | uint8(Ns_VirtualFrameStatusFlg),
      | uint8(Ns_IncompleteFrameCntFlg),
      | uint8(Ns_OverflowCntFlg),
      | uint16(Ns_FrameBufferSize),
      | double(Ns_SampleTime)
      mask prompts: Ns_DeviceID "Device:"; Ns_ChannelNum "Channel number:"; Ns_FrameID "Frame ID:"; Ns_IsVirtualFrame "Belong to a virtual frame"; Ns_RoleInVirtualFrame "Position in virtual frame:"; Ns_HeaderFrameID "Header frame ID:"; Ns_VirtualFrameStatusFlg "Current virtural frame status output"; Ns_IncompleteFrameCntFlg "Incomplete virtual frame count output"; Ns_OverflowCntFlg "Overflow count output"; Ns_FrameBufferSize "Frame buffer size:"; Ns_SampleTime "Sample time:"
      mask init:
      | NSTC297CANReceive_callback('portlabels');
      mask TypeOptions Ns_DeviceID: General Control Unit Gen2 | ADAS Control Unit Gen2
      mask TypeOptions Ns_ChannelNum: 0 | 1 | 2 | 3 | 4 | 5
      mask Callback Ns_IsVirtualFrame: NSTC297CANReceive_callback('Belong to a virtual frame');
      mask TypeOptions Ns_RoleInVirtualFrame: Header Frame | Data Frame | Trailer Frame
      mask Callback Ns_RoleInVirtualFrame: NSTC297CANReceive_callback('Position in virtual frame');
      mask Display: color('blue');text(0.02,0.9,'NovSteeds TC297','horizontalAlignment','left');color('blue');text(0.5,0.7,'CAN Receive','horizontalAlignment','center');color('black');text(0.5,0.6,'Channel: 4','horizontalAlignment','center');text(0.5,0.5,'ID: 667','horizontalAlignment','center');text(0.5,0.4,'Virtual Frame: No','horizontalAlignment','center');port_label('output',1, 'RemainderCnt');port_label('output',2, 'Msg');
  Acc_DisplaySig : Outport
  wires:
  S-Function11/2 -> CAN Unpack2/1
  CAN Unpack2/10 -> Bus Creator/10  "AEB_tips"
  CAN Unpack2/9 -> Bus Creator/9  "AEB_Switch_Status"
  CAN Unpack2/11 -> Bus Creator/11  "ICA_HMI_Txt_Disp"
  CAN Unpack2/8 -> Bus Creator/8  "AEB_Fault_Status"
  CAN Unpack2/12 -> Bus Creator/12  "RVVACC_Vehiclespeed_request_type"
  CAN Unpack2/7 -> Bus Creator/7  "AEB_Alert_Req"
  CAN Unpack2/13 -> Bus Creator/13  "TJA_status_icon"
  CAN Unpack2/6 -> Bus Creator/6  "ACC_Vehicle_Icon_Display"
  CAN Unpack2/5 -> Bus Creator/5  "ACC_Set_Speed_Display"
  CAN Unpack2/4 -> Bus Creator/4  "ACC_Pop_Up_Message"
  CAN Unpack2/3 -> Bus Creator/3  "ACC_Desired_Set_Speed"
  CAN Unpack2/2 -> Bus Creator/2  "ACC_DesiredHeadway_Icon_Basic"
  CAN Unpack2/1 -> Bus Creator/1  "ACC_DesiredHeadway_Display"
  Bus Creator/1 -> Acc_DisplaySig/1
